simulink model "PID_Regler2test"  (Simulink 7.6)
settings: Solver=ode45  SolverMode=SingleTasking  StartTime=0.0  StopTime=10000  RelTol=1e-3
libraries: simulink x1, modelsimlib x1
settings Model: Creator=azafar  LastModifiedBy=Stefan
settings OptimizationCC: InlineParams=on
settings DebuggingCC: FcnCallInpInsideContextMsg=Enable All
settings HardwareCC: ProdHWDeviceType=ASIC/FPGA->ASIC/FPGA  TargetIntDivRoundTo=Zero  TargetEndianess=LittleEndian  TargetHWDeviceType=MATLAB Host  ProdEqTarget=off

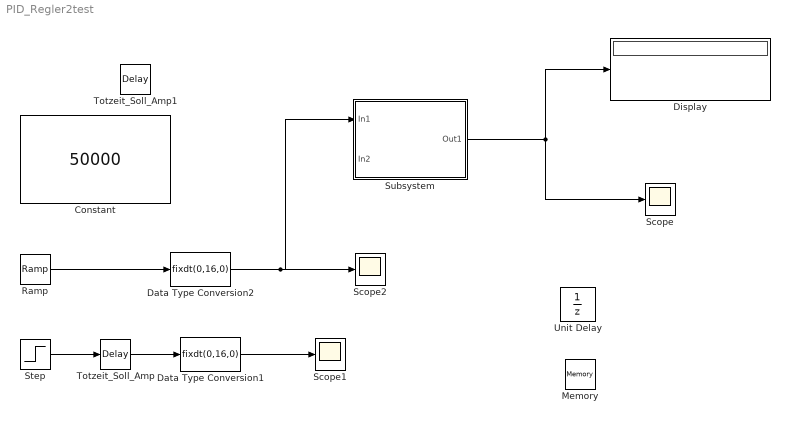
== system PID_Regler2test ==
  Constant : Constant  Value=50000  OutDataTypeStr=fixdt(0,16,0)  SampleTime=1
  Data Type Conversion1 : DataTypeConversion  OutDataTypeStr=fixdt(0,16,0)  SampleTime=1
  Data Type Conversion2 : DataTypeConversion  OutDataTypeStr=fixdt(0,16,0)  SampleTime=1
  Display : Display
      settings: Format=decimal (Stored Integer)
  Memory : Memory
  Ramp : simulink/Sources/Ramp  SystemSampleTime=-1  slope=1  start=1  X0=10
  Scope : Scope
  Scope1 : Scope
      settings: SaveName=ScopeData3
  Scope2 : Scope
      settings: YMin=0  YMax=70000  SaveName=ScopeData4
  Step : Step  Time=0.0001  Before=1  After=2  SampleTime=1
  Subsystem : Subsystem
  Totzeit_Soll_Amp : TransportDelay  DelayTime=0.5*10^(-5)
  Totzeit_Soll_Amp1 : TransportDelay  DelayTime=0.5*10^(-5)
  Unit Delay : UnitDelay  SampleTime=-1
  wires:
  Subsystem/1(Out1) -> Display/1, Scope/1
  Data Type Conversion1/1 -> Scope1/1
  Ramp/1 -> Data Type Conversion2/1
  Step/1 -> Totzeit_Soll_Amp/1
  Totzeit_Soll_Amp/1 -> Data Type Conversion1/1
  Data Type Conversion2/1 -> Subsystem/1(In1), Scope2/1

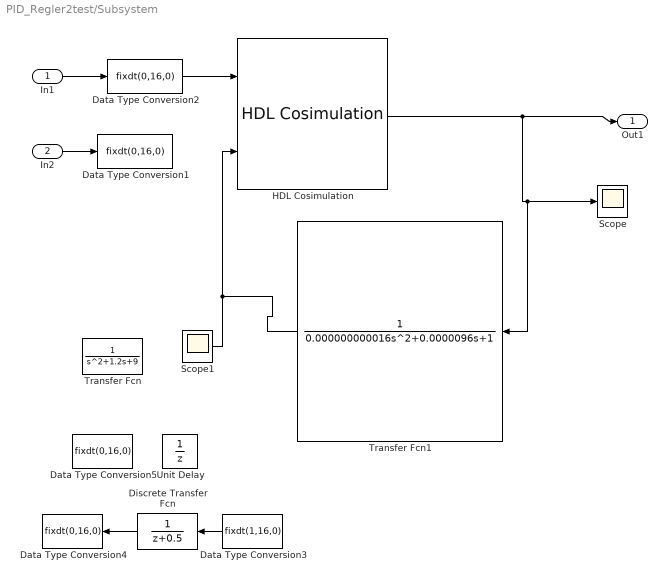
== system PID_Regler2test/Subsystem ==
  In1 : Inport  OutDataTypeStr=fixdt(0,16,0)
  In2 : Inport  Port=2  OutDataTypeStr=fixdt(0,16,0)
  Data Type Conversion1 : DataTypeConversion  OutDataTypeStr=fixdt(0,16,0)
  Data Type Conversion2 : DataTypeConversion  OutDataTypeStr=fixdt(0,16,0)  SampleTime=1
  Data Type Conversion3 : DataTypeConversion  OutDataTypeStr=fixdt(1,16,0)  SampleTime=1
  Data Type Conversion4 : DataTypeConversion  OutDataTypeStr=fixdt(0,16,0)  SampleTime=1
  Data Type Conversion5 : DataTypeConversion  OutDataTypeStr=fixdt(0,16,0)  SampleTime=1
  Discrete Transfer Fcn : DiscreteTransferFcn  StateDataTypeStr=fixdt(1,16,0)
  HDL Cosimulation : modelsimlib/HDL Cosimulation  DialogController=hdllinkddg.CoSimBlockDialog  SystemSampleTime=-1  PortPaths=/pi_controller_and_feed_forward_tb/dut/data_w_i;/pi_controller_and_feed_forward_tb/dut/data_y_i;/pi_controller_and_feed_forward_tb/dut/data_u_o  PortModes=[1 1 2 ]  PortTimes=[-1,-1,10]  PortSigns=[-1 -1 -1 ]  PortFracLengths=[0,0,0]  CommLocal=on  CommSharedMemory=on  CommPortNumber=4449  CommShowInfo=on  ClockPaths=/pi_controller_and_feed_forward_tb/dut/clk_i  ClockModes=[2 ]  ClockTimes=[2]  TclPreSimCommand="echo \"Running pi_controller_and_feed_forward in Simulink.\""  TclPostSimCommand="echo \"Done\""  TimingMode=Tick  TimingScaleFactor=1  idxCellArray={'UNUSED_VAR'}  CosimBypass=Full Simulation  AllowDirectFeedthrough=on  ProductName=EDA Simulator Link MQ  RunAutoTimescale=off  HdlClocks=0
  Scope : Scope
      settings: TimeRange=50000  YMin=0  YMax=35000
  Scope1 : Scope
      settings: YMin=0  YMax=35000  SaveName=ScopeData2
  Transfer Fcn : TransferFcn  Denominator=[1 1.2 9]
  Transfer Fcn1 : TransferFcn  Denominator=[0.000000000016 0.0000096 1]
  Unit Delay : UnitDelay
  Out1 : Outport  OutDataTypeStr=fixdt(0,16,0)
  wires:
  In2/1 -> Data Type Conversion1/1
  In1/1 -> Data Type Conversion2/1
  Data Type Conversion2/1 -> HDL Cosimulation/1
  HDL Cosimulation/1 -> Out1/1, Scope/1, Transfer Fcn1/1
  Discrete Transfer Fcn/1 -> Data Type Conversion4/1
  Data Type Conversion3/1 -> Discrete Transfer Fcn/1
  Transfer Fcn1/1 -> HDL Cosimulation/2, Scope1/1
